simulink model "Oppgave1a"  (R2021b)
settings: Solver=FixedStepAuto  StartTime=0.0  StopTime=10  FixedStep=1e-3  RelTol=1e-3
model workspace (MATLAB code in the model file):
  | m1 = 5000; %kg
  | 
  | 
  | %%fluids
  | Cd = 0.6;
  | Ad1 = 9e-6; %m^2
  | Ad2 = 5e-6; %m^2
  | Ad3 = Ad1;
  | Ad4 = Ad2;
  | 
  | Rho = 875; %kg/m^2
  | Beta = 830% MPa
  | 
  | V0 = 1e-3; %m^3
  | 
  | %% Starting values
  | x1 = 0; %m
  | 
  | x1dot = 0;
  | 
  | p0 = 0;
undefined symbols (not defined in the file): X, Y, Z
libraries: fl_lib x14, nesl_utility x7, sm_lib x6, sh_lib x3
settings Model: Creator=Philip  LastModifiedBy=student

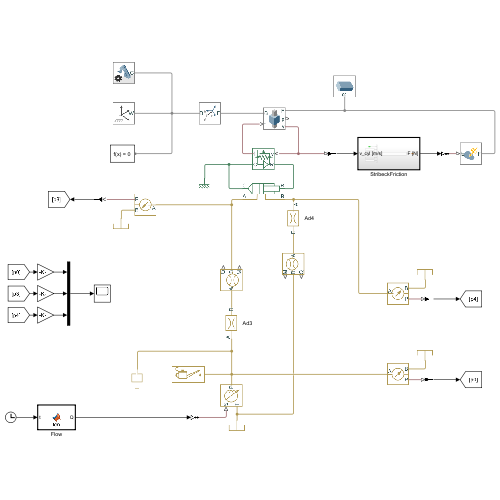
[thumbnail: Simulink's stored preview of the top-level diagram]
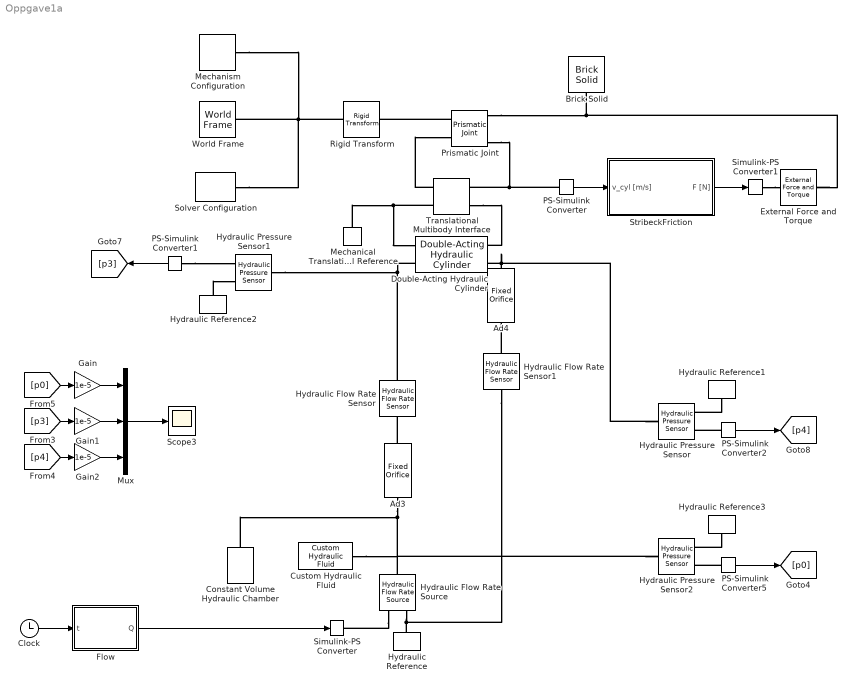
== system Oppgave1a ==
  Ad3 : sh_lib/Orifices/Fixed Orifice  area=Ad3 m^2  C_d=Cd  lam_spec=1  B_lam=0.999  Re_cr=12  q_specify=off  q_priority=None  q=0.001 m^3/s  q_nominal_specify=off  q_nominal_unit=m^3/s  q_nominal_value=1  p_specify=off  p_priority=None  p=0 Pa  p_nominal_specify=off  p_nominal_unit=Pa  p_nominal_value=1
      settings: SourceProductBaseCode=SH  InternalSimscapePortConfiguration="{\"Bottom\":[],\"Left\":[{\"id\":\"A\",\"label\":\"A\",\"type\":\"foundation.hydraulic.hydraulic\"}],\"Right\":[{\"id\":\"B\",\"label\":\"B\",\"type\":\"foundation.hydraulic.hydraulic\"}],\"Top\":[]}"
  Ad4 : sh_lib/Orifices/Fixed Orifice  area=Ad4 m^2  C_d=Cd  lam_spec=1  B_lam=0.999  Re_cr=12  q_specify=off  q_priority=None  q=0.001 m^3/s  q_nominal_specify=off  q_nominal_unit=m^3/s  q_nominal_value=1  p_specify=off  p_priority=None  p=0 Pa  p_nominal_specify=off  p_nominal_unit=Pa  p_nominal_value=1
      settings: SourceProductBaseCode=SH  InternalSimscapePortConfiguration="{\"Bottom\":[],\"Left\":[{\"id\":\"A\",\"label\":\"A\",\"type\":\"foundation.hydraulic.hydraulic\"}],\"Right\":[{\"id\":\"B\",\"label\":\"B\",\"type\":\"foundation.hydraulic.hydraulic\"}],\"Top\":[]}"
  Brick Solid : sm_lib/Body Elements/Brick Solid  GraphicAmbientColor=[0.15 0.15 0.15 1.0]  BasedOnType=Mass  BrickDimensions=[1 1 1]  BrickDimensionUnits=m  CenterOfMass=[0 0 0]  CenterOfMassUnits=m  GraphicDiffuseColor=[0.5 0.5 0.5]  Density=1000  DensityUnits=kg/m^3  DoExposeReferenceFrame=on  GraphicEmissiveColor=[0.0 0.0 0.0 1.0]  ExportEntireGeometry=off  SerializedFrames=<Frames/>  MarkerShape=Sphere  MarkerSize=10  GraphicType=FromGeometry  InertiaType=CalculateFromGeometry  Mass=3000  MassUnits=kg  MomentsOfInertia=[1 1 1]  MomentsOfInertiaUnits=kg*m^2  GraphicOpacity=1.0  ProductsOfInertia=[0 0 0]  ProductsOfInertiaUnits=kg*m^2  GraphicShininess=75  GraphicSpecularColor=[0.5 0.5 0.5 1.0]  GraphicVisPropType=SimpleVisualProperties
  Clock : Clock
  Constant Volume Hydraulic Chamber : fl_lib/Hydraulic/Hydraulic Elements/Constant Volume Hydraulic Chamber  ch_sp=foundation.enum.chamberGeometry.volume  wall_type=foundation.enum.chamber_spec.rigid  ch_volume=V0 m^3  d_in=1e-2 m  length=1 m  pr_r_coef=1.2e-12 m/Pa  time_const=0.01 s  k_sh=1.4  pressure_specify=off  pressure_priority=High  pressure=0 Pa  pressure_nominal_specify=off  pressure_nominal_unit=Pa  pressure_nominal_value=1  diameter_incr_specify=off  diameter_incr_priority=High  diameter_incr=0 m  diameter_incr_nominal_specify=off  diameter_incr_nominal_unit=m  diameter_incr_nominal_value=1  flow_rate_specify=off  flow_rate_priority=None  flow_rate=0.001 m^3/s  flow_rate_nominal_specify=off  flow_rate_nominal_unit=m^3/s  flow_rate_nominal_value=1
      settings: SourceProductBaseCode=SS  InternalSimscapePortConfiguration="{\"Bottom\":[],\"Left\":[{\"id\":\"A\",\"label\":\"\",\"type\":\"foundation.hydraulic.hydraulic\"}],\"Right\":[],\"Top\":[]}"
  Custom Hydraulic Fluid : fl_lib/Hydraulic/Hydraulic Utilities/Custom Hydraulic Fluid  density=Rho kg/m^3  viscosity_kin=18e-6 m^2/s  bulk=1.200 MPa  alpha=0.005  range_error=2
      settings: SourceProductBaseCode=SS  InternalSimscapePortConfiguration="{\"Bottom\":[],\"Left\":[],\"Right\":[{\"id\":\"G\",\"label\":\"\",\"type\":\"foundation.hydraulic.hydraulic\"}],\"Top\":[]}"
  Double-Acting Hydraulic Cylinder : sh_lib/Hydraulic Cylinders/Double-Acting Hydraulic Cylinder  area_A=pi*0.042^2/4 m^2  area_B=pi*(0.042^2-0.03^2)/4 m^2  stroke=1.6 m  dead_vol_A=1e-5 m^3  dead_vol_B=1e-5 m^3  k_sh=1.4  or=sh.cylinders.enum.MechOrientationTranslational.Positive  stiff=1e6 N/m  D=150 N/(m/s)  hardstop_model=1  transition=0.1 mm  displacement_spec=foundation.enum.DisplacementSpec.Calculate  init_pos=0 m  init_pressure_A=0 Pa  init_pressure_B=0 Pa
      settings: SourceProductBaseCode=SH  InternalSimscapePortConfiguration="{\"Bottom\":[],\"Left\":[{\"id\":\"C\",\"label\":\"C\",\"type\":\"foundation.mechanical.translational.translational\"},{\"id\":\"A\",\"label\":\"A\",\"type\":\"foundation.hydraulic.hydraulic\"}],\"Right\":[{\"id\":\"R\",\"label\":\"R\",\"type\":\"foundation.mechanical.translational.translational\"},{\"id\":\"B\",\"label\":\"B\",\"type\":\"foundation.hydraulic.hydraulic\"}],\"Top\":[]}"
  External Force and Torque : sm_lib/Forces and Torques/External Force and Torque  ForceResolutionFrame=AttachedFrame  EnableForceX=off  EnableForceY=off  EnableForceZ=on  EnableForce=off  TorqueResolutionFrame=AttachedFrame  EnableTorqueX=off  EnableTorqueY=off  EnableTorqueZ=off  EnableTorque=off
  Flow : MATLAB Function  TreatAsAtomicUnit=on
  Gain : Gain  Gain=1e-5
  Gain1 : Gain  Gain=1e-5
  Gain2 : Gain  Gain=1e-5
  Hydraulic Flow Rate Sensor : fl_lib/Hydraulic/Hydraulic Sensors/Hydraulic Flow Rate Sensor
  Hydraulic Flow Rate Sensor1 : fl_lib/Hydraulic/Hydraulic Sensors/Hydraulic Flow Rate Sensor
  Hydraulic Flow Rate Source : fl_lib/Hydraulic/Hydraulic Sources/Hydraulic Flow Rate Source
      settings: SourceProductBaseCode=SS  InternalSimscapePortConfiguration="{\"Bottom\":[],\"Left\":[{\"id\":\"P\",\"label\":\"P\",\"type\":\"foundation.hydraulic.hydraulic\"}],\"Right\":[{\"id\":\"S\",\"label\":\"S\",\"type\":\"input\"},{\"id\":\"T\",\"label\":\"T\",\"type\":\"foundation.hydraulic.hydraulic\"}],\"Top\":[]}"
  Hydraulic Pressure Sensor : fl_lib/Hydraulic/Hydraulic Sensors/Hydraulic Pressure Sensor
  Hydraulic Pressure Sensor1 : fl_lib/Hydraulic/Hydraulic Sensors/Hydraulic Pressure Sensor
  Hydraulic Pressure Sensor2 : fl_lib/Hydraulic/Hydraulic Sensors/Hydraulic Pressure Sensor
  Hydraulic Reference{,1..3} (4 alike) : fl_lib/Hydraulic/Hydraulic Elements/Hydraulic Reference
  Mechanical Translational Reference : fl_lib/Mechanical/Translational Elements/Mechanical Translational Reference
  Mechanism Configuration : sm_lib/Utilities/Mechanism Configuration  UniformGravity=Constant  GravityVector=[0 0 -9.80665]  GravityUnits=m/s^2  LinearizationDelta=0.001  JointModeTransitionNonlinearIterations=2
  Mux : Mux  Inputs=3
  PS-Simulink Converter{,1..2,5} (4 alike) : nesl_utility/PS-Simulink Converter  PhysicalDomain=network_engine_domain  SubClassName=ps_output  LeftPortType=input  RightPortType=output  PseudoPeriodic=off  Frequencies=[]  Unit=inherit  AffineConversion=off
      settings: SourceProductBaseCode=PW,SS
  Prismatic Joint : sm_lib/Joints/Prismatic Joint  JointMode=Normal  SenseConstraintForce=off  SenseConstraintForceX=off  SenseConstraintForceY=off  SenseConstraintForceZ=off  SenseConstraintTorque=off  SenseConstraintTorqueX=off  SenseConstraintTorqueY=off  SenseConstraintTorqueZ=off  SenseTotalForce=off  SenseTotalForceX=off  SenseTotalForceY=off  SenseTotalForceZ=off  SenseTotalTorque=off  SenseTotalTorqueX=off  SenseTotalTorqueY=off  SenseTotalTorqueZ=off  CompositeWrenchDir=FollowerOnBase  CompositeWrenchFrame=BaseFrame  EquilibriumPosition=0  EquilibriumPositionUnits=m  SpringStiffness=0  SpringStiffnessUnits=N/m  DampingCoefficient=0  DampingCoefficientUnits=N/(m/s)  TorqueActuationMode=InputTorque  MotionActuationMode=ComputedMotion  SensePosition=on  SenseVelocity=on  SenseAcceleration=off  SenseTorqueForce=off  SenseLowerLimitTorqueForce=off  SenseUpperLimitTorqueForce=off  LowerLimitSpecify=off  LowerLimitBound=-1  LowerLimitBoundUnits=m  LowerLimitStiffness=1e6  LowerLimitStiffnessUnits=N/m  LowerLimitDamping=1e3  LowerLimitDampingUnits=N/(m/s)  LowerLimitTransitionRegionWidth=1e-4  LowerLimitTransitionRegionWidthUnits=m  UpperLimitSpecify=off  UpperLimitBound=1  UpperLimitBoundUnits=m  UpperLimitStiffness=1e6  UpperLimitStiffnessUnits=N/m  UpperLimitDamping=1e3  UpperLimitDampingUnits=N/(m/s)  UpperLimitTransitionRegionWidth=1e-4  UpperLimitTransitionRegionWidthUnits=m  PositionTargetSpecify=on  PositionTargetPriority=High  PositionTargetValue=0.2  PositionTargetValueUnits=m  VelocityTargetSpecify=on  VelocityTargetPriority=High  VelocityTargetValue=0  VelocityTargetValueUnits=m/s
  Rigid Transform : sm_lib/Frames and Transforms/Rigid Transform  TranslationMethod=None  TranslationStandardOffset=0  TranslationLengthUnit=m  TranslationStandardAxis=+Z  TranslationCartesianOffset=[0 0 0]  TranslationROffset=0  TranslationROffsetUnits=m  TranslationZOffset=0  TranslationZOffsetUnits=m  TranslationThetaOffset=0  TranslationThetaOffsetUnits=deg  RotationMethod=RotationSequence  RotationAngleUnits=deg  RotationStandardAxis=+Z  RotationAngle=0.0  RotationArbitraryAxis=[0 0 1]  FollAlignAxisA=+X  BaseAlignAxisA=+Y  FollAlignAxisB=+Y  BaseAlignAxisB=+Z  RotationSequenceAxes=FollowerAxes  RotationSequence=XYX  RotationSequenceAngles=[0 90 0]  RotationSequenceAnglesUnits=deg  RotationMatrix=[1 0 0; 0 1 0; 0 0 1]
  Scope3 : Scope
  Simulink-PS Converter : nesl_utility/Simulink-PS Converter  PhysicalDomain=network_engine_domain  SubClassName=ps_input  LeftPortType=input  RightPortType=output  PseudoPeriodic=off  Frequencies=[]  NoiseDistribution=none  NoiseParameters=[]  Unit=1  AffineConversion=off  FilteringAndDerivatives=filter  SimscapeFilterOrder=2  InputFilterTimeConstant=0.001  UdotUserProvided=0
      settings: SourceProductBaseCode=PW,SS
  Simulink-PS Converter1 : nesl_utility/Simulink-PS Converter  PhysicalDomain=network_engine_domain  SubClassName=ps_input  LeftPortType=input  RightPortType=output  PseudoPeriodic=off  Frequencies=[]  NoiseDistribution=none  NoiseParameters=[]  Unit=1  AffineConversion=off  FilteringAndDerivatives=filter  SimscapeFilterOrder=2  InputFilterTimeConstant=0.001  UdotUserProvided=0
      settings: SourceProductBaseCode=PW,SS
  Solver Configuration : nesl_utility/Solver Configuration  PhysicalDomain=network_engine_domain  SubClassName=solver  LeftPortType=input  RightPortType=generic  Tones=[]  Harmonics=[]  SimulateNoise=off  Profile=off  UseLocalSampling=off  EnableSwitchedLinearOptims=on  FrequencyDomain=off  UseCCode=off  RelTol=0.001  AbsTol=1e-06  MinStep=1e-09  ToWorkspace=off  RevertToSquareIcSolve=off  NumHomotopyIterations=100  PhasorMode=off  PhasorModeNumHarmonics=1  DoDC=off  ResidualTolerance=1e-09  UseLocalSolver=off  LocalSolverChoice=NE_BACKWARD_EULER_ADVANCER  LocalSolverSampleTime=0.001  DoFixedCost=off  MaxNonlinIter=3  MaxModeIter=2  ComputeImpulses=off  ImpulseIterations=2  LinearAlgebra=auto  EquationFormulation=NE_TIME_EF  DelaysMemoryBudget=1024  AutomaticFiltering=on  FilteringTimeConstant=0.001  PartitionStorageMethod=AS_NEEDED  PartitionMemoryBudget=1024  PartitionMethod=ROBUST
      settings: SourceProductBaseCode=PW,SS
  StribeckFriction : Subsystem  TreatAsAtomicUnit=on
  Translational Multibody Interface : fl_lib/Mechanical/Multibody Interfaces/Translational Multibody Interface
      settings: SourceProductBaseCode=SS
  World Frame : sm_lib/Frames and Transforms/World Frame
  wires:
  Clock/1 -> Flow/1(t)
  Flow/1(Q) -> Simulink-PS Converter/1
  StribeckFriction/1(F [N]) -> Simulink-PS Converter1/1
  PS-Simulink Converter/1 -> StribeckFriction/1(v_cyl [m/s])
  PS-Simulink Converter5/1 -> [p0]
  PS-Simulink Converter1/1 -> [p3]
  PS-Simulink Converter2/1 -> [p4]
  [p0] -> Gain/1
  Mux/1 -> Scope3/1
  Gain/1 -> Mux/1
  [p3] -> Gain1/1
  Gain1/1 -> Mux/2
  [p4] -> Gain2/1
  Gain2/1 -> Mux/3
  connections:
  Mechanism Configuration/RConn1 -- Rigid Transform/LConn1 -- Solver Configuration/RConn1 -- World Frame/RConn1
  Hydraulic Reference/LConn1 -- Hydraulic Flow Rate Sensor1/RConn2 -- Hydraulic Flow Rate Source/RConn2
  Hydraulic Flow Rate Source/RConn1 -- Simulink-PS Converter/RConn1
  Hydraulic Flow Rate Source/LConn1 -- Custom Hydraulic Fluid/RConn1 -- Hydraulic Pressure Sensor2/LConn1 -- Ad3/LConn1 -- Constant Volume Hydraulic Chamber/LConn1
  Ad4/LConn1 -- Hydraulic Pressure Sensor/LConn1 -- Double-Acting Hydraulic Cylinder/RConn2
  Translational Multibody Interface/LConn2 -- Double-Acting Hydraulic Cylinder/LConn1 -- Mechanical Translational Reference/LConn1
  Translational Multibody Interface/RConn2 -- Double-Acting Hydraulic Cylinder/RConn1
  Prismatic Joint/LConn1 -- Rigid Transform/RConn1
  Translational Multibody Interface/LConn1 -- Prismatic Joint/LConn2
  Prismatic Joint/RConn1 -- External Force and Torque/RConn1 -- Brick Solid/RConn1
  Simulink-PS Converter1/RConn1 -- External Force and Torque/LConn1
  Double-Acting Hydraulic Cylinder/LConn2 -- Hydraulic Flow Rate Sensor/RConn2 -- Hydraulic Pressure Sensor1/LConn1
  Hydraulic Flow Rate Sensor1/LConn1 -- Ad4/RConn1
  Prismatic Joint/RConn3 -- PS-Simulink Converter/LConn1 -- Translational Multibody Interface/RConn1
  Hydraulic Reference1/LConn1 -- Hydraulic Pressure Sensor/RConn1
  PS-Simulink Converter2/LConn1 -- Hydraulic Pressure Sensor/RConn2
  Ad3/RConn1 -- Hydraulic Flow Rate Sensor/LConn1
  Hydraulic Reference2/LConn1 -- Hydraulic Pressure Sensor1/RConn1
  PS-Simulink Converter1/LConn1 -- Hydraulic Pressure Sensor1/RConn2
  Hydraulic Reference3/LConn1 -- Hydraulic Pressure Sensor2/RConn1
  PS-Simulink Converter5/LConn1 -- Hydraulic Pressure Sensor2/RConn2

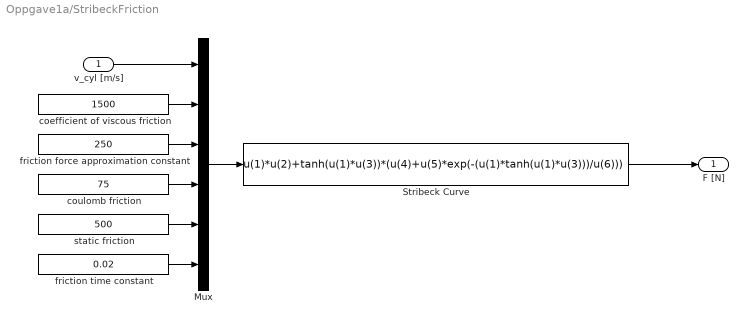
== system Oppgave1a/StribeckFriction ==
  v_cyl [m/s] : Inport
  Mux : Mux  Inputs=6
  Stribeck Curve : Fcn  Expr=u(1)*u(2)+tanh(u(1)*u(3))*(u(4)+u(5)*exp(-(u(1)*tanh(u(1)*u(3)))/u(6)))
  "coefficient of viscous friction " : Constant  Value=1500
  coulomb friction : Constant  Value=75
  friction force approximation constant : Constant  Value=250
  friction time constant : Constant  Value=0.02
  static friction : Constant  Value=500
  F [N] : Outport  VectorParamsAs1DForOutWhenUnconnected=off
  wires:
  friction time constant/1 -> Mux/6
  v_cyl [m/s]/1 -> Mux/1
  static friction/1 -> Mux/5
  "coefficient of viscous friction "/1 -> Mux/2
  friction force approximation constant/1 -> Mux/3
  Mux/1 -> Stribeck Curve/1
  coulomb friction/1 -> Mux/4
  Stribeck Curve/1 -> F [N]/1

== matlab function Oppgave1a/Flow ==
  data: t input; Q output
function Q = fcn(t)
Qmax = 25*1/60e3; %L/min
tramp = 0.25;
t1 = 0.25;
t2 = 1.25;
t3 = 1.5;

if t<t1
    Q = Qmax/tramp * t;
elseif t<t2
    Q = Qmax;
elseif t<t3
    Q = -Qmax/tramp * (t-t2) + Qmax;
else
    Q = 0;
end
